simulink model "Beam_simulation_FA23"  (R2019a)
settings: Solver=ode45  StartTime=0.0  StopTime=10  FixedStep=5e-7  MaxStep=0.01  RelTol=1e-3  EnableMultiTasking=on
undefined symbols (not defined in the file or in its folder): A, B, C, D
settings Model: Creator=vnatara2  LastModifiedBy=OyunaA
settings DataIOCC: LimitDataPoints=on  SaveFormat=Array  SignalLoggingSaveFormat=ModelDataLogs  SaveOutput=off  SaveTime=off  ReturnWorkspaceOutputs=off
settings OptimizationCC: ExpressionDepthLimit=2147483647  InitFltsAndDblsToZero=on  LifeSpan=inf
settings DebuggingCC: SaveWithParameterizedLinksMsg=none  UnderspecifiedInitializationDetection=Classic  MergeDetectMultiDrivingBlocksExec=none  SolverPrmCheckMsg=warning  FcnCallInpInsideContextMsg=warning  StateNameClashWarn=warning  PregeneratedLibrarySubsystemCodeDiagnostic=none  SFUnexpectedBacktrackingDiag=warning  SFNoUnconditionalDefaultTransitionDiag=warning  SFExecutionAtInitializationDiag=none  ArithmeticOperatorsInVariantConditions=warning
settings HardwareCC: ProdBitPerPointer=32  ProdBitPerSizeT=32  ProdBitPerPtrDiffT=32  ProdLargestAtomicFloat=None  ProdIntDivRoundTo=Undefined  ProdEndianess=Unspecified  ProdWordSize=32  ProdHWDeviceType=32-bit Generic
settings ModelReferenceCC: PropagateSignalLabelsOutOfModel=off
settings SFSimCC: SimUseLocalCustomCode=off
settings RTWCC: RTWUseLocalCustomCode=off
settings CodeAppCC: StateflowObjectComments=on
settings GRTTargetCC: TargetFcnLib=ansi_tfl_tmw.mat  TargetLangStandard=C89/C90 (ANSI)  GeneratePreprocessorConditionals=Disable all  CombineOutputUpdateFcns=off  GRTInterface=on
settings ConfigComp: CovMetricSettings=dw  CovHtmlReporting=on  CovSaveCumulativeToWorkspaceVar=on  CovSaveSingleToWorkspaceVar=on  CovExternalEMLEnable=off  CovSFcnEnable=off

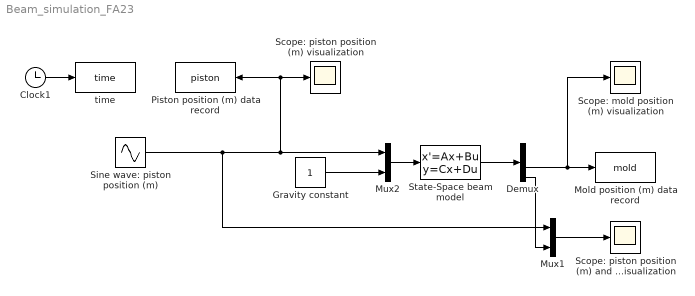
== system Beam_simulation_FA23 ==
  "Clock1 " : Clock
  Demux : Demux
  Gravity constant : Constant
  Mold position (m) data record : ToWorkspace  VariableName=mold  SampleTime=0.002
      settings: MaxDataPoints=1250
  Mux1 : Mux  Inputs=2
  Mux2 : Mux  Inputs=2
  Piston position (m) data record : ToWorkspace  VariableName=piston  SampleTime=0.002
      settings: MaxDataPoints=1250
  Scope: mold position (m) visualization : Scope
  Scope: piston position (m) visualization : Scope
  Scope: piston position (m) and mold velocity (m/s) visualization : Scope
  "Sine wave: piston position (m) " : Sin  Amplitude=10/1000  Frequency=2*pi*4.6  SampleTime=0
  State-Space beam model : StateSpace  A=A  B=B  C=C  D=D  InitialCondition=0
  time : ToWorkspace  VariableName=time  SampleTime=0.002
      settings: MaxDataPoints=1250
  wires:
  Mux2/1 -> State-Space beam model/1
  "Clock1 "/1 -> time/1
  State-Space beam model/1 -> Demux/1
  Demux/3 -> Scope: mold position (m) visualization/1, Mold position (m) data record/1
  "Sine wave: piston position (m) "/1 -> Mux1/1, Mux2/1, Scope: piston position (m) visualization/1, Piston position (m) data record/1
  Demux/4 -> Mux1/2
  Mux1/1 -> Scope: piston position (m) and mold velocity (m/s) visualization/1
  Gravity constant/1 -> Mux2/2
